simulink model "battery_pack_72v"  (R2020a)
settings: Solver=ode23t  StartTime=0.0  StopTime=5  RelTol=1e-3
libraries: fl_lib x1674, nesl_utility x2
(part 1 of 13)
settings Model: Creator=SIDD N  LastModifiedBy=SIDD N

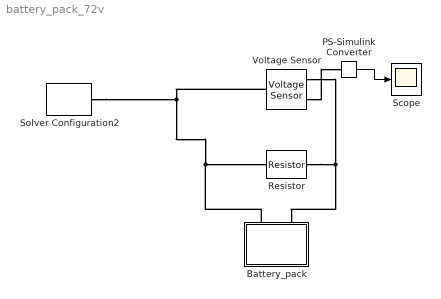
== system battery_pack_72v ==
  Battery_pack : Subsystem
      mask Display: image('$imagefile'); % Use "Edit Image" on toolstrip to change.
  PS-Simulink Converter : nesl_utility/PS-Simulink Converter  PhysicalDomain=network_engine_domain  SubClassName=ps_output  LeftPortType=input  RightPortType=output  PseudoPeriodic=off  Frequencies=[]  Unit=inherit  AffineConversion=off
  Resistor : fl_lib/Electrical/Electrical Elements/Resistor  R=10000 Ohm  i_specify=off  i_priority=None  i=0 A  i_nominal_specify=off  i_nominal_unit=A  i_nominal_value=1  v_specify=off  v_priority=None  v=0 V  v_nominal_specify=off  v_nominal_unit=V  v_nominal_value=1
  Scope : Scope
  Solver Configuration2 : nesl_utility/Solver Configuration  PhysicalDomain=network_engine_domain  SubClassName=solver  LeftPortType=input  RightPortType=generic  Tones=[]  Harmonics=[]  SimulateNoise=off  Profile=off  UseLocalSampling=off  EnableSwitchedLinearOptims=on  FrequencyDomain=off  UseCCode=off  RelTol=0.001  AbsTol=1e-06  MinStep=1e-09  ToWorkspace=off  RevertToSquareIcSolve=off  NumHomotopyIterations=100  PhasorMode=off  PhasorModeNumHarmonics=1  DoDC=off  ResidualTolerance=1e-09  UseLocalSolver=off  LocalSolverChoice=NE_BACKWARD_EULER_ADVANCER  LocalSolverSampleTime=1e-7  DoFixedCost=off  MaxNonlinIter=3  MaxModeIter=2  LinearAlgebra=Sparse  EquationFormulation=NE_TIME_EF  DelaysMemoryBudget=1024  AutomaticFiltering=on  FilteringTimeConstant=0.001  PartitionStorageMethod=AS_NEEDED  PartitionMemoryBudget=1024  PartitionMethod=FAST
  Voltage Sensor : fl_lib/Electrical/Electrical Sensors/Voltage Sensor
  wires:
  PS-Simulink Converter/1 -> Scope/1
  connections:
  Voltage Sensor/RConn1 -- PS-Simulink Converter/LConn1
  Voltage Sensor/LConn1 -- Solver Configuration2/RConn1 -- Battery_pack/LConn1 -- Resistor/LConn1
  Voltage Sensor/RConn2 -- Resistor/RConn1 -- Battery_pack/LConn2

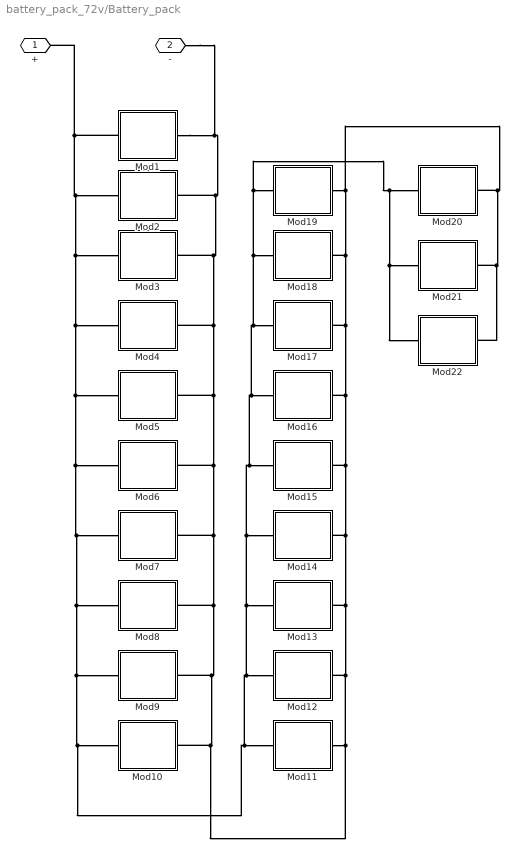
== system battery_pack_72v/Battery_pack ==
  Mod1 : Subsystem
      mask Display: image('C:\Users\SIDD N\Desktop\Screenshot 2020-11-21 19581dwqdq9.png'); % Use "Edit Image" on toolstrip to change.
  Mod10 : Subsystem
      mask Display: image('C:\Users\SIDD N\Desktop\Screenshot 2020-11-21 19581dwqdq9.png'); % Use "Edit Image" on toolstrip to change.
  Mod11 : Subsystem
      mask Display: image('C:\Users\SIDD N\Desktop\Screenshot 2020-11-21 19581dwqdq9.png'); % Use "Edit Image" on toolstrip to change.
  Mod12 : Subsystem
      mask Display: image('C:\Users\SIDD N\Desktop\Screenshot 2020-11-21 19581dwqdq9.png'); % Use "Edit Image" on toolstrip to change.
  Mod13 : Subsystem
      mask Display: image('C:\Users\SIDD N\Desktop\Screenshot 2020-11-21 19581dwqdq9.png'); % Use "Edit Image" on toolstrip to change.
  Mod14 : Subsystem
      mask Display: image('C:\Users\SIDD N\Desktop\Screenshot 2020-11-21 19581dwqdq9.png'); % Use "Edit Image" on toolstrip to change.
  Mod15 : Subsystem
      mask Display: image('C:\Users\SIDD N\Desktop\Screenshot 2020-11-21 19581dwqdq9.png'); % Use "Edit Image" on toolstrip to change.
  Mod16 : Subsystem
      mask Display: image('C:\Users\SIDD N\Desktop\Screenshot 2020-11-21 19581dwqdq9.png'); % Use "Edit Image" on toolstrip to change.
  Mod17 : Subsystem
      mask Display: image('C:\Users\SIDD N\Desktop\Screenshot 2020-11-21 19581dwqdq9.png'); % Use "Edit Image" on toolstrip to change.
  Mod18 : Subsystem
      mask Display: image('C:\Users\SIDD N\Desktop\Screenshot 2020-11-21 19581dwqdq9.png'); % Use "Edit Image" on toolstrip to change.
  Mod19 : Subsystem
      mask Display: image('C:\Users\SIDD N\Desktop\Screenshot 2020-11-21 19581dwqdq9.png'); % Use "Edit Image" on toolstrip to change.
  Mod2 : Subsystem
      mask Display: image('C:\Users\SIDD N\Desktop\Screenshot 2020-11-21 19581dwqdq9.png'); % Use "Edit Image" on toolstrip to change.
  Mod20 : Subsystem
      mask Display: image('C:\Users\SIDD N\Desktop\Screenshot 2020-11-21 19581dwqdq9.png'); % Use "Edit Image" on toolstrip to change.
  Mod21 : Subsystem
      mask Display: image('C:\Users\SIDD N\Desktop\Screenshot 2020-11-21 19581dwqdq9.png'); % Use "Edit Image" on toolstrip to change.
  Mod22 : Subsystem
      mask Display: image('C:\Users\SIDD N\Desktop\Screenshot 2020-11-21 19581dwqdq9.png'); % Use "Edit Image" on toolstrip to change.
  Mod3 : Subsystem
      mask Display: image('C:\Users\SIDD N\Desktop\Screenshot 2020-11-21 19581dwqdq9.png'); % Use "Edit Image" on toolstrip to change.
  Mod4 : Subsystem
      mask Display: image('C:\Users\SIDD N\Desktop\Screenshot 2020-11-21 19581dwqdq9.png'); % Use "Edit Image" on toolstrip to change.
  Mod5 : Subsystem
      mask Display: image('C:\Users\SIDD N\Desktop\Screenshot 2020-11-21 19581dwqdq9.png'); % Use "Edit Image" on toolstrip to change.
  Mod6 : Subsystem
      mask Display: image('C:\Users\SIDD N\Desktop\Screenshot 2020-11-21 19581dwqdq9.png'); % Use "Edit Image" on toolstrip to change.
  Mod7 : Subsystem
      mask Display: image('C:\Users\SIDD N\Desktop\Screenshot 2020-11-21 19581dwqdq9.png'); % Use "Edit Image" on toolstrip to change.
  Mod8 : Subsystem
      mask Display: image('C:\Users\SIDD N\Desktop\Screenshot 2020-11-21 19581dwqdq9.png'); % Use "Edit Image" on toolstrip to change.
  Mod9 : Subsystem
      mask Display: image('C:\Users\SIDD N\Desktop\Screenshot 2020-11-21 19581dwqdq9.png'); % Use "Edit Image" on toolstrip to change.
  + : PMIOPort  Side=Left
  - : PMIOPort  Port=2  Side=Left
  connections:
  Mod19/RConn1 -- Mod12/RConn1 -- Mod11/RConn1 -- Mod10/RConn1 -- Mod9/RConn1 -- Mod6/RConn1 -- Mod4/RConn1 -- Mod3/RConn1 -- -/RConn1 -- Mod1/RConn1 -- Mod2/RConn1 -- Mod5/RConn1 -- Mod7/RConn1 -- Mod8/RConn1 -- Mod13/RConn1 -- Mod14/RConn1 -- Mod15/RConn1 -- Mod16/RConn1 -- Mod17/RConn1 -- Mod18/RConn1 -- Mod22/RConn1 -- Mod21/RConn1 -- Mod20/RConn1
  Mod22/LConn1 -- Mod21/LConn1 -- Mod20/LConn1 -- Mod19/LConn1 -- Mod18/LConn1 -- Mod17/LConn1 -- Mod16/LConn1 -- Mod15/LConn1 -- Mod14/LConn1 -- Mod13/LConn1 -- Mod12/LConn1 -- Mod11/LConn1 -- Mod10/LConn1 -- Mod9/LConn1 -- Mod8/LConn1 -- Mod7/LConn1 -- Mod6/LConn1 -- Mod5/LConn1 -- Mod4/LConn1 -- Mod3/LConn1 -- Mod2/LConn1 -- +/RConn1 -- Mod1/LConn1

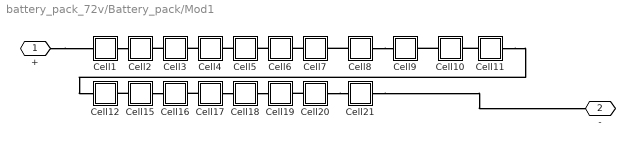
== system battery_pack_72v/Battery_pack/Mod1 ==
  Cell1 : Subsystem
  Cell10 : Subsystem
  Cell11 : Subsystem
  Cell12 : Subsystem
  Cell15 : Subsystem
  Cell16 : Subsystem
  Cell17 : Subsystem
  Cell18 : Subsystem
  Cell19 : Subsystem
  Cell2 : Subsystem
  Cell20 : Subsystem
  Cell21 : Subsystem
  Cell3 : Subsystem
  Cell4 : Subsystem
  Cell5 : Subsystem
  Cell6 : Subsystem
  Cell7 : Subsystem
  Cell8 : Subsystem
  Cell9 : Subsystem
  + : PMIOPort  Side=Left
  - : PMIOPort  Port=2  Side=Right
  connections:
  Cell15/RConn1 -- Cell16/LConn1
  Cell11/LConn1 -- Cell10/RConn1
  Cell8/LConn1 -- Cell7/RConn1
  Cell20/LConn1 -- Cell19/RConn1
  Cell7/LConn1 -- Cell6/RConn1
  Cell17/LConn1 -- Cell16/RConn1
  Cell20/RConn1 -- Cell21/LConn1
  Cell17/RConn1 -- Cell18/LConn1
  Cell3/LConn1 -- Cell2/RConn1
  Cell5/LConn1 -- Cell4/RConn1
  Cell18/RConn1 -- Cell19/LConn1
  Cell8/RConn1 -- Cell9/LConn1
  Cell15/LConn1 -- Cell12/RConn1
  Cell4/LConn1 -- Cell3/RConn1
  Cell11/RConn1 -- Cell12/LConn1
  Cell10/LConn1 -- Cell9/RConn1
  Cell6/LConn1 -- Cell5/RConn1
  Cell1/RConn1 -- Cell2/LConn1
  Cell21/RConn1 -- -/RConn1
  +/RConn1 -- Cell1/LConn1

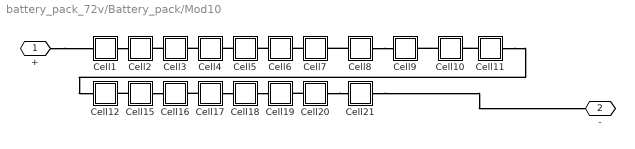
== system battery_pack_72v/Battery_pack/Mod10 ==
  Cell1 : Subsystem
  Cell10 : Subsystem
  Cell11 : Subsystem
  Cell12 : Subsystem
  Cell15 : Subsystem
  Cell16 : Subsystem
  Cell17 : Subsystem
  Cell18 : Subsystem
  Cell19 : Subsystem
  Cell2 : Subsystem
  Cell20 : Subsystem
  Cell21 : Subsystem
  Cell3 : Subsystem
  Cell4 : Subsystem
  Cell5 : Subsystem
  Cell6 : Subsystem
  Cell7 : Subsystem
  Cell8 : Subsystem
  Cell9 : Subsystem
  + : PMIOPort  Side=Left
  - : PMIOPort  Port=2  Side=Right
  connections:
  +/RConn1 -- Cell1/LConn1
  Cell21/RConn1 -- -/RConn1
  Cell1/RConn1 -- Cell2/LConn1
  Cell6/LConn1 -- Cell5/RConn1
  Cell10/LConn1 -- Cell9/RConn1
  Cell11/RConn1 -- Cell12/LConn1
  Cell4/LConn1 -- Cell3/RConn1
  Cell15/LConn1 -- Cell12/RConn1
  Cell8/RConn1 -- Cell9/LConn1
  Cell18/RConn1 -- Cell19/LConn1
  Cell5/LConn1 -- Cell4/RConn1
  Cell3/LConn1 -- Cell2/RConn1
  Cell17/RConn1 -- Cell18/LConn1
  Cell20/RConn1 -- Cell21/LConn1
  Cell17/LConn1 -- Cell16/RConn1
  Cell7/LConn1 -- Cell6/RConn1
  Cell20/LConn1 -- Cell19/RConn1
  Cell8/LConn1 -- Cell7/RConn1
  Cell11/LConn1 -- Cell10/RConn1
  Cell15/RConn1 -- Cell16/LConn1

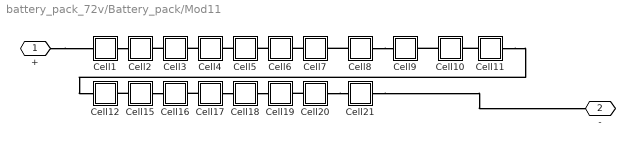
== system battery_pack_72v/Battery_pack/Mod11 ==
  Cell1 : Subsystem
  Cell10 : Subsystem
  Cell11 : Subsystem
  Cell12 : Subsystem
  Cell15 : Subsystem
  Cell16 : Subsystem
  Cell17 : Subsystem
  Cell18 : Subsystem
  Cell19 : Subsystem
  Cell2 : Subsystem
  Cell20 : Subsystem
  Cell21 : Subsystem
  Cell3 : Subsystem
  Cell4 : Subsystem
  Cell5 : Subsystem
  Cell6 : Subsystem
  Cell7 : Subsystem
  Cell8 : Subsystem
  Cell9 : Subsystem
  + : PMIOPort  Side=Left
  - : PMIOPort  Port=2  Side=Right
  connections:
  +/RConn1 -- Cell1/LConn1
  Cell21/RConn1 -- -/RConn1
  Cell1/RConn1 -- Cell2/LConn1
  Cell6/LConn1 -- Cell5/RConn1
  Cell10/LConn1 -- Cell9/RConn1
  Cell11/RConn1 -- Cell12/LConn1
  Cell4/LConn1 -- Cell3/RConn1
  Cell15/LConn1 -- Cell12/RConn1
  Cell8/RConn1 -- Cell9/LConn1
  Cell18/RConn1 -- Cell19/LConn1
  Cell5/LConn1 -- Cell4/RConn1
  Cell3/LConn1 -- Cell2/RConn1
  Cell17/RConn1 -- Cell18/LConn1
  Cell20/RConn1 -- Cell21/LConn1
  Cell17/LConn1 -- Cell16/RConn1
  Cell7/LConn1 -- Cell6/RConn1
  Cell20/LConn1 -- Cell19/RConn1
  Cell8/LConn1 -- Cell7/RConn1
  Cell11/LConn1 -- Cell10/RConn1
  Cell15/RConn1 -- Cell16/LConn1

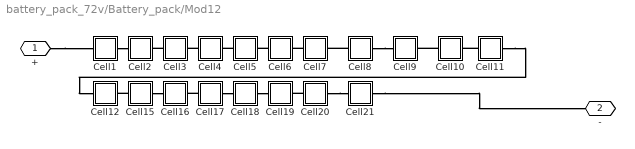
== system battery_pack_72v/Battery_pack/Mod12 ==
  Cell1 : Subsystem
  Cell10 : Subsystem
  Cell11 : Subsystem
  Cell12 : Subsystem
  Cell15 : Subsystem
  Cell16 : Subsystem
  Cell17 : Subsystem
  Cell18 : Subsystem
  Cell19 : Subsystem
  Cell2 : Subsystem
  Cell20 : Subsystem
  Cell21 : Subsystem
  Cell3 : Subsystem
  Cell4 : Subsystem
  Cell5 : Subsystem
  Cell6 : Subsystem
  Cell7 : Subsystem
  Cell8 : Subsystem
  Cell9 : Subsystem
  + : PMIOPort  Side=Left
  - : PMIOPort  Port=2  Side=Right
  connections:
  Cell15/RConn1 -- Cell16/LConn1
  Cell11/LConn1 -- Cell10/RConn1
  Cell8/LConn1 -- Cell7/RConn1
  Cell20/LConn1 -- Cell19/RConn1
  Cell7/LConn1 -- Cell6/RConn1
  Cell17/LConn1 -- Cell16/RConn1
  Cell20/RConn1 -- Cell21/LConn1
  Cell17/RConn1 -- Cell18/LConn1
  Cell3/LConn1 -- Cell2/RConn1
  Cell5/LConn1 -- Cell4/RConn1
  Cell18/RConn1 -- Cell19/LConn1
  Cell8/RConn1 -- Cell9/LConn1
  Cell15/LConn1 -- Cell12/RConn1
  Cell4/LConn1 -- Cell3/RConn1
  Cell11/RConn1 -- Cell12/LConn1
  Cell10/LConn1 -- Cell9/RConn1
  Cell6/LConn1 -- Cell5/RConn1
  Cell1/RConn1 -- Cell2/LConn1
  Cell21/RConn1 -- -/RConn1
  +/RConn1 -- Cell1/LConn1

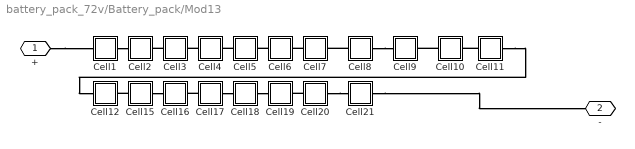
== system battery_pack_72v/Battery_pack/Mod13 ==
  Cell1 : Subsystem
  Cell10 : Subsystem
  Cell11 : Subsystem
  Cell12 : Subsystem
  Cell15 : Subsystem
  Cell16 : Subsystem
  Cell17 : Subsystem
  Cell18 : Subsystem
  Cell19 : Subsystem
  Cell2 : Subsystem
  Cell20 : Subsystem
  Cell21 : Subsystem
  Cell3 : Subsystem
  Cell4 : Subsystem
  Cell5 : Subsystem
  Cell6 : Subsystem
  Cell7 : Subsystem
  Cell8 : Subsystem
  Cell9 : Subsystem
  + : PMIOPort  Side=Left
  - : PMIOPort  Port=2  Side=Right
  connections:
  Cell15/RConn1 -- Cell16/LConn1
  Cell11/LConn1 -- Cell10/RConn1
  Cell8/LConn1 -- Cell7/RConn1
  Cell20/LConn1 -- Cell19/RConn1
  Cell7/LConn1 -- Cell6/RConn1
  Cell17/LConn1 -- Cell16/RConn1
  Cell20/RConn1 -- Cell21/LConn1
  Cell17/RConn1 -- Cell18/LConn1
  Cell3/LConn1 -- Cell2/RConn1
  Cell5/LConn1 -- Cell4/RConn1
  Cell18/RConn1 -- Cell19/LConn1
  Cell8/RConn1 -- Cell9/LConn1
  Cell15/LConn1 -- Cell12/RConn1
  Cell4/LConn1 -- Cell3/RConn1
  Cell11/RConn1 -- Cell12/LConn1
  Cell10/LConn1 -- Cell9/RConn1
  Cell6/LConn1 -- Cell5/RConn1
  Cell1/RConn1 -- Cell2/LConn1
  Cell21/RConn1 -- -/RConn1
  +/RConn1 -- Cell1/LConn1

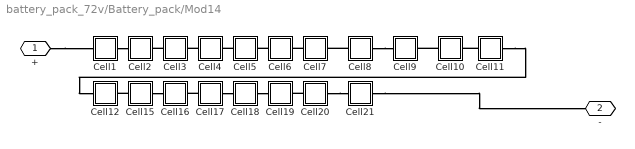
== system battery_pack_72v/Battery_pack/Mod14 ==
  Cell1 : Subsystem
  Cell10 : Subsystem
  Cell11 : Subsystem
  Cell12 : Subsystem
  Cell15 : Subsystem
  Cell16 : Subsystem
  Cell17 : Subsystem
  Cell18 : Subsystem
  Cell19 : Subsystem
  Cell2 : Subsystem
  Cell20 : Subsystem
  Cell21 : Subsystem
  Cell3 : Subsystem
  Cell4 : Subsystem
  Cell5 : Subsystem
  Cell6 : Subsystem
  Cell7 : Subsystem
  Cell8 : Subsystem
  Cell9 : Subsystem
  + : PMIOPort  Side=Left
  - : PMIOPort  Port=2  Side=Right
  connections:
  +/RConn1 -- Cell1/LConn1
  Cell21/RConn1 -- -/RConn1
  Cell1/RConn1 -- Cell2/LConn1
  Cell6/LConn1 -- Cell5/RConn1
  Cell10/LConn1 -- Cell9/RConn1
  Cell11/RConn1 -- Cell12/LConn1
  Cell4/LConn1 -- Cell3/RConn1
  Cell15/LConn1 -- Cell12/RConn1
  Cell8/RConn1 -- Cell9/LConn1
  Cell18/RConn1 -- Cell19/LConn1
  Cell5/LConn1 -- Cell4/RConn1
  Cell3/LConn1 -- Cell2/RConn1
  Cell17/RConn1 -- Cell18/LConn1
  Cell20/RConn1 -- Cell21/LConn1
  Cell17/LConn1 -- Cell16/RConn1
  Cell7/LConn1 -- Cell6/RConn1
  Cell20/LConn1 -- Cell19/RConn1
  Cell8/LConn1 -- Cell7/RConn1
  Cell11/LConn1 -- Cell10/RConn1
  Cell15/RConn1 -- Cell16/LConn1

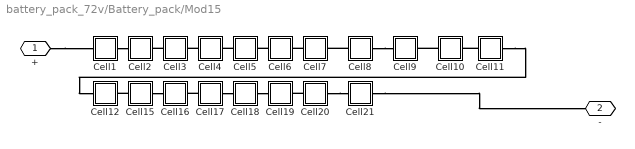
== system battery_pack_72v/Battery_pack/Mod15 ==
  Cell1 : Subsystem
  Cell10 : Subsystem
  Cell11 : Subsystem
  Cell12 : Subsystem
  Cell15 : Subsystem
  Cell16 : Subsystem
  Cell17 : Subsystem
  Cell18 : Subsystem
  Cell19 : Subsystem
  Cell2 : Subsystem
  Cell20 : Subsystem
  Cell21 : Subsystem
  Cell3 : Subsystem
  Cell4 : Subsystem
  Cell5 : Subsystem
  Cell6 : Subsystem
  Cell7 : Subsystem
  Cell8 : Subsystem
  Cell9 : Subsystem
  + : PMIOPort  Side=Left
  - : PMIOPort  Port=2  Side=Right
  connections:
  Cell15/RConn1 -- Cell16/LConn1
  Cell11/LConn1 -- Cell10/RConn1
  Cell8/LConn1 -- Cell7/RConn1
  Cell20/LConn1 -- Cell19/RConn1
  Cell7/LConn1 -- Cell6/RConn1
  Cell17/LConn1 -- Cell16/RConn1
  Cell20/RConn1 -- Cell21/LConn1
  Cell17/RConn1 -- Cell18/LConn1
  Cell3/LConn1 -- Cell2/RConn1
  Cell5/LConn1 -- Cell4/RConn1
  Cell18/RConn1 -- Cell19/LConn1
  Cell8/RConn1 -- Cell9/LConn1
  Cell15/LConn1 -- Cell12/RConn1
  Cell4/LConn1 -- Cell3/RConn1
  Cell11/RConn1 -- Cell12/LConn1
  Cell10/LConn1 -- Cell9/RConn1
  Cell6/LConn1 -- Cell5/RConn1
  Cell1/RConn1 -- Cell2/LConn1
  Cell21/RConn1 -- -/RConn1
  +/RConn1 -- Cell1/LConn1

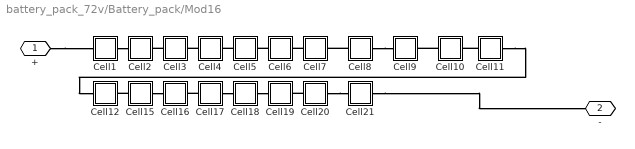
== system battery_pack_72v/Battery_pack/Mod16 ==
  Cell1 : Subsystem
  Cell10 : Subsystem
  Cell11 : Subsystem
  Cell12 : Subsystem
  Cell15 : Subsystem
  Cell16 : Subsystem
  Cell17 : Subsystem
  Cell18 : Subsystem
  Cell19 : Subsystem
  Cell2 : Subsystem
  Cell20 : Subsystem
  Cell21 : Subsystem
  Cell3 : Subsystem
  Cell4 : Subsystem
  Cell5 : Subsystem
  Cell6 : Subsystem
  Cell7 : Subsystem
  Cell8 : Subsystem
  Cell9 : Subsystem
  + : PMIOPort  Side=Left
  - : PMIOPort  Port=2  Side=Right
  connections:
  +/RConn1 -- Cell1/LConn1
  Cell21/RConn1 -- -/RConn1
  Cell1/RConn1 -- Cell2/LConn1
  Cell6/LConn1 -- Cell5/RConn1
  Cell10/LConn1 -- Cell9/RConn1
  Cell11/RConn1 -- Cell12/LConn1
  Cell4/LConn1 -- Cell3/RConn1
  Cell15/LConn1 -- Cell12/RConn1
  Cell8/RConn1 -- Cell9/LConn1
  Cell18/RConn1 -- Cell19/LConn1
  Cell5/LConn1 -- Cell4/RConn1
  Cell3/LConn1 -- Cell2/RConn1
  Cell17/RConn1 -- Cell18/LConn1
  Cell20/RConn1 -- Cell21/LConn1
  Cell17/LConn1 -- Cell16/RConn1
  Cell7/LConn1 -- Cell6/RConn1
  Cell20/LConn1 -- Cell19/RConn1
  Cell8/LConn1 -- Cell7/RConn1
  Cell11/LConn1 -- Cell10/RConn1
  Cell15/RConn1 -- Cell16/LConn1

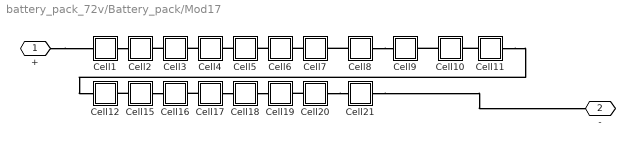
== system battery_pack_72v/Battery_pack/Mod17 ==
  Cell1 : Subsystem
  Cell10 : Subsystem
  Cell11 : Subsystem
  Cell12 : Subsystem
  Cell15 : Subsystem
  Cell16 : Subsystem
  Cell17 : Subsystem
  Cell18 : Subsystem
  Cell19 : Subsystem
  Cell2 : Subsystem
  Cell20 : Subsystem
  Cell21 : Subsystem
  Cell3 : Subsystem
  Cell4 : Subsystem
  Cell5 : Subsystem
  Cell6 : Subsystem
  Cell7 : Subsystem
  Cell8 : Subsystem
  Cell9 : Subsystem
  + : PMIOPort  Side=Left
  - : PMIOPort  Port=2  Side=Right
  connections:
  Cell15/RConn1 -- Cell16/LConn1
  Cell11/LConn1 -- Cell10/RConn1
  Cell8/LConn1 -- Cell7/RConn1
  Cell20/LConn1 -- Cell19/RConn1
  Cell7/LConn1 -- Cell6/RConn1
  Cell17/LConn1 -- Cell16/RConn1
  Cell20/RConn1 -- Cell21/LConn1
  Cell17/RConn1 -- Cell18/LConn1
  Cell3/LConn1 -- Cell2/RConn1
  Cell5/LConn1 -- Cell4/RConn1
  Cell18/RConn1 -- Cell19/LConn1
  Cell8/RConn1 -- Cell9/LConn1
  Cell15/LConn1 -- Cell12/RConn1
  Cell4/LConn1 -- Cell3/RConn1
  Cell11/RConn1 -- Cell12/LConn1
  Cell10/LConn1 -- Cell9/RConn1
  Cell6/LConn1 -- Cell5/RConn1
  Cell1/RConn1 -- Cell2/LConn1
  Cell21/RConn1 -- -/RConn1
  +/RConn1 -- Cell1/LConn1

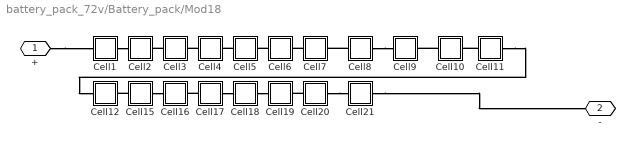
== system battery_pack_72v/Battery_pack/Mod18 ==
  Cell1 : Subsystem
  Cell10 : Subsystem
  Cell11 : Subsystem
  Cell12 : Subsystem
  Cell15 : Subsystem
  Cell16 : Subsystem
  Cell17 : Subsystem
  Cell18 : Subsystem
  Cell19 : Subsystem
  Cell2 : Subsystem
  Cell20 : Subsystem
  Cell21 : Subsystem
  Cell3 : Subsystem
  Cell4 : Subsystem
  Cell5 : Subsystem
  Cell6 : Subsystem
  Cell7 : Subsystem
  Cell8 : Subsystem
  Cell9 : Subsystem
  + : PMIOPort  Side=Left
  - : PMIOPort  Port=2  Side=Right
  connections:
  +/RConn1 -- Cell1/LConn1
  Cell21/RConn1 -- -/RConn1
  Cell1/RConn1 -- Cell2/LConn1
  Cell6/LConn1 -- Cell5/RConn1
  Cell10/LConn1 -- Cell9/RConn1
  Cell11/RConn1 -- Cell12/LConn1
  Cell4/LConn1 -- Cell3/RConn1
  Cell15/LConn1 -- Cell12/RConn1
  Cell8/RConn1 -- Cell9/LConn1
  Cell18/RConn1 -- Cell19/LConn1
  Cell5/LConn1 -- Cell4/RConn1
  Cell3/LConn1 -- Cell2/RConn1
  Cell17/RConn1 -- Cell18/LConn1
  Cell20/RConn1 -- Cell21/LConn1
  Cell17/LConn1 -- Cell16/RConn1
  Cell7/LConn1 -- Cell6/RConn1
  Cell20/LConn1 -- Cell19/RConn1
  Cell8/LConn1 -- Cell7/RConn1
  Cell11/LConn1 -- Cell10/RConn1
  Cell15/RConn1 -- Cell16/LConn1

== system battery_pack_72v/Battery_pack/Mod19 ==
  Cell1 : Subsystem
  Cell10 : Subsystem
  Cell11 : Subsystem
  Cell12 : Subsystem
  Cell15 : Subsystem
  Cell16 : Subsystem
  Cell17 : Subsystem
  Cell18 : Subsystem
  Cell19 : Subsystem
  Cell2 : Subsystem
  Cell20 : Subsystem
  Cell21 : Subsystem
  Cell3 : Subsystem
  Cell4 : Subsystem
  Cell5 : Subsystem
  Cell6 : Subsystem
  Cell7 : Subsystem
  Cell8 : Subsystem
  Cell9 : Subsystem
  + : PMIOPort  Side=Left
  - : PMIOPort  Port=2  Side=Right
  connections:
  Cell15/RConn1 -- Cell16/LConn1
  Cell11/LConn1 -- Cell10/RConn1
  Cell8/LConn1 -- Cell7/RConn1
  Cell20/LConn1 -- Cell19/RConn1
  Cell7/LConn1 -- Cell6/RConn1
  Cell17/LConn1 -- Cell16/RConn1
  Cell20/RConn1 -- Cell21/LConn1
  Cell17/RConn1 -- Cell18/LConn1
  Cell3/LConn1 -- Cell2/RConn1
  Cell5/LConn1 -- Cell4/RConn1
  Cell18/RConn1 -- Cell19/LConn1
  Cell8/RConn1 -- Cell9/LConn1
  Cell15/LConn1 -- Cell12/RConn1
  Cell4/LConn1 -- Cell3/RConn1
  Cell11/RConn1 -- Cell12/LConn1
  Cell10/LConn1 -- Cell9/RConn1
  Cell6/LConn1 -- Cell5/RConn1
  Cell1/RConn1 -- Cell2/LConn1
  Cell21/RConn1 -- -/RConn1
  +/RConn1 -- Cell1/LConn1

== system battery_pack_72v/Battery_pack/Mod2 ==
  Cell1 : Subsystem
  Cell10 : Subsystem
  Cell11 : Subsystem
  Cell12 : Subsystem
  Cell15 : Subsystem
  Cell16 : Subsystem
  Cell17 : Subsystem
  Cell18 : Subsystem
  Cell19 : Subsystem
  Cell2 : Subsystem
  Cell20 : Subsystem
  Cell21 : Subsystem
  Cell3 : Subsystem
  Cell4 : Subsystem
  Cell5 : Subsystem
  Cell6 : Subsystem
  Cell7 : Subsystem
  Cell8 : Subsystem
  Cell9 : Subsystem
  + : PMIOPort  Side=Left
  - : PMIOPort  Port=2  Side=Right
  connections:
  +/RConn1 -- Cell1/LConn1
  Cell21/RConn1 -- -/RConn1
  Cell1/RConn1 -- Cell2/LConn1
  Cell6/LConn1 -- Cell5/RConn1
  Cell10/LConn1 -- Cell9/RConn1
  Cell11/RConn1 -- Cell12/LConn1
  Cell4/LConn1 -- Cell3/RConn1
  Cell15/LConn1 -- Cell12/RConn1
  Cell8/RConn1 -- Cell9/LConn1
  Cell18/RConn1 -- Cell19/LConn1
  Cell5/LConn1 -- Cell4/RConn1
  Cell3/LConn1 -- Cell2/RConn1
  Cell17/RConn1 -- Cell18/LConn1
  Cell20/RConn1 -- Cell21/LConn1
  Cell17/LConn1 -- Cell16/RConn1
  Cell7/LConn1 -- Cell6/RConn1
  Cell20/LConn1 -- Cell19/RConn1
  Cell8/LConn1 -- Cell7/RConn1
  Cell11/LConn1 -- Cell10/RConn1
  Cell15/RConn1 -- Cell16/LConn1

== system battery_pack_72v/Battery_pack/Mod20 ==
  Cell1 : Subsystem
  Cell10 : Subsystem
  Cell11 : Subsystem
  Cell12 : Subsystem
  Cell15 : Subsystem
  Cell16 : Subsystem
  Cell17 : Subsystem
  Cell18 : Subsystem
  Cell19 : Subsystem
  Cell2 : Subsystem
  Cell20 : Subsystem
  Cell21 : Subsystem
  Cell3 : Subsystem
  Cell4 : Subsystem
  Cell5 : Subsystem
  Cell6 : Subsystem
  Cell7 : Subsystem
  Cell8 : Subsystem
  Cell9 : Subsystem
  + : PMIOPort  Side=Left
  - : PMIOPort  Port=2  Side=Right
  connections:
  +/RConn1 -- Cell1/LConn1
  Cell21/RConn1 -- -/RConn1
  Cell1/RConn1 -- Cell2/LConn1
  Cell6/LConn1 -- Cell5/RConn1
  Cell10/LConn1 -- Cell9/RConn1
  Cell11/RConn1 -- Cell12/LConn1
  Cell4/LConn1 -- Cell3/RConn1
  Cell15/LConn1 -- Cell12/RConn1
  Cell8/RConn1 -- Cell9/LConn1
  Cell18/RConn1 -- Cell19/LConn1
  Cell5/LConn1 -- Cell4/RConn1
  Cell3/LConn1 -- Cell2/RConn1
  Cell17/RConn1 -- Cell18/LConn1
  Cell20/RConn1 -- Cell21/LConn1
  Cell17/LConn1 -- Cell16/RConn1
  Cell7/LConn1 -- Cell6/RConn1
  Cell20/LConn1 -- Cell19/RConn1
  Cell8/LConn1 -- Cell7/RConn1
  Cell11/LConn1 -- Cell10/RConn1
  Cell15/RConn1 -- Cell16/LConn1

== system battery_pack_72v/Battery_pack/Mod21 ==
  Cell1 : Subsystem
  Cell10 : Subsystem
  Cell11 : Subsystem
  Cell12 : Subsystem
  Cell15 : Subsystem
  Cell16 : Subsystem
  Cell17 : Subsystem
  Cell18 : Subsystem
  Cell19 : Subsystem
  Cell2 : Subsystem
  Cell20 : Subsystem
  Cell21 : Subsystem
  Cell3 : Subsystem
  Cell4 : Subsystem
  Cell5 : Subsystem
  Cell6 : Subsystem
  Cell7 : Subsystem
  Cell8 : Subsystem
  Cell9 : Subsystem
  + : PMIOPort  Side=Left
  - : PMIOPort  Port=2  Side=Right
  connections:
  Cell15/RConn1 -- Cell16/LConn1
  Cell11/LConn1 -- Cell10/RConn1
  Cell8/LConn1 -- Cell7/RConn1
  Cell20/LConn1 -- Cell19/RConn1
  Cell7/LConn1 -- Cell6/RConn1
  Cell17/LConn1 -- Cell16/RConn1
  Cell20/RConn1 -- Cell21/LConn1
  Cell17/RConn1 -- Cell18/LConn1
  Cell3/LConn1 -- Cell2/RConn1
  Cell5/LConn1 -- Cell4/RConn1
  Cell18/RConn1 -- Cell19/LConn1
  Cell8/RConn1 -- Cell9/LConn1
  Cell15/LConn1 -- Cell12/RConn1
  Cell4/LConn1 -- Cell3/RConn1
  Cell11/RConn1 -- Cell12/LConn1
  Cell10/LConn1 -- Cell9/RConn1
  Cell6/LConn1 -- Cell5/RConn1
  Cell1/RConn1 -- Cell2/LConn1
  Cell21/RConn1 -- -/RConn1
  +/RConn1 -- Cell1/LConn1

== system battery_pack_72v/Battery_pack/Mod22 ==
  Cell1 : Subsystem
  Cell10 : Subsystem
  Cell11 : Subsystem
  Cell12 : Subsystem
  Cell15 : Subsystem
  Cell16 : Subsystem
  Cell17 : Subsystem
  Cell18 : Subsystem
  Cell19 : Subsystem
  Cell2 : Subsystem
  Cell20 : Subsystem
  Cell21 : Subsystem
  Cell3 : Subsystem
  Cell4 : Subsystem
  Cell5 : Subsystem
  Cell6 : Subsystem
  Cell7 : Subsystem
  Cell8 : Subsystem
  Cell9 : Subsystem
  + : PMIOPort  Side=Left
  - : PMIOPort  Port=2  Side=Right
  connections:
  +/RConn1 -- Cell1/LConn1
  Cell21/RConn1 -- -/RConn1
  Cell1/RConn1 -- Cell2/LConn1
  Cell6/LConn1 -- Cell5/RConn1
  Cell10/LConn1 -- Cell9/RConn1
  Cell11/RConn1 -- Cell12/LConn1
  Cell4/LConn1 -- Cell3/RConn1
  Cell15/LConn1 -- Cell12/RConn1
  Cell8/RConn1 -- Cell9/LConn1
  Cell18/RConn1 -- Cell19/LConn1
  Cell5/LConn1 -- Cell4/RConn1
  Cell3/LConn1 -- Cell2/RConn1
  Cell17/RConn1 -- Cell18/LConn1
  Cell20/RConn1 -- Cell21/LConn1
  Cell17/LConn1 -- Cell16/RConn1
  Cell7/LConn1 -- Cell6/RConn1
  Cell20/LConn1 -- Cell19/RConn1
  Cell8/LConn1 -- Cell7/RConn1
  Cell11/LConn1 -- Cell10/RConn1
  Cell15/RConn1 -- Cell16/LConn1

== system battery_pack_72v/Battery_pack/Mod3 ==
  Cell1 : Subsystem
  Cell10 : Subsystem
  Cell11 : Subsystem
  Cell12 : Subsystem
  Cell15 : Subsystem
  Cell16 : Subsystem
  Cell17 : Subsystem
  Cell18 : Subsystem
  Cell19 : Subsystem
  Cell2 : Subsystem
  Cell20 : Subsystem
  Cell21 : Subsystem
  Cell3 : Subsystem
  Cell4 : Subsystem
  Cell5 : Subsystem
  Cell6 : Subsystem
  Cell7 : Subsystem
  Cell8 : Subsystem
  Cell9 : Subsystem
  + : PMIOPort  Side=Left
  - : PMIOPort  Port=2  Side=Right
  connections:
  Cell15/RConn1 -- Cell16/LConn1
  Cell11/LConn1 -- Cell10/RConn1
  Cell8/LConn1 -- Cell7/RConn1
  Cell20/LConn1 -- Cell19/RConn1
  Cell7/LConn1 -- Cell6/RConn1
  Cell17/LConn1 -- Cell16/RConn1
  Cell20/RConn1 -- Cell21/LConn1
  Cell17/RConn1 -- Cell18/LConn1
  Cell3/LConn1 -- Cell2/RConn1
  Cell5/LConn1 -- Cell4/RConn1
  Cell18/RConn1 -- Cell19/LConn1
  Cell8/RConn1 -- Cell9/LConn1
  Cell15/LConn1 -- Cell12/RConn1
  Cell4/LConn1 -- Cell3/RConn1
  Cell11/RConn1 -- Cell12/LConn1
  Cell10/LConn1 -- Cell9/RConn1
  Cell6/LConn1 -- Cell5/RConn1
  Cell1/RConn1 -- Cell2/LConn1
  Cell21/RConn1 -- -/RConn1
  +/RConn1 -- Cell1/LConn1

== system battery_pack_72v/Battery_pack/Mod4 ==
  Cell1 : Subsystem
  Cell10 : Subsystem
  Cell11 : Subsystem
  Cell12 : Subsystem
  Cell15 : Subsystem
  Cell16 : Subsystem
  Cell17 : Subsystem
  Cell18 : Subsystem
  Cell19 : Subsystem
  Cell2 : Subsystem
  Cell20 : Subsystem
  Cell21 : Subsystem
  Cell3 : Subsystem
  Cell4 : Subsystem
  Cell5 : Subsystem
  Cell6 : Subsystem
  Cell7 : Subsystem
  Cell8 : Subsystem
  Cell9 : Subsystem
  + : PMIOPort  Side=Left
  - : PMIOPort  Port=2  Side=Right
  connections:
  +/RConn1 -- Cell1/LConn1
  Cell21/RConn1 -- -/RConn1
  Cell1/RConn1 -- Cell2/LConn1
  Cell6/LConn1 -- Cell5/RConn1
  Cell10/LConn1 -- Cell9/RConn1
  Cell11/RConn1 -- Cell12/LConn1
  Cell4/LConn1 -- Cell3/RConn1
  Cell15/LConn1 -- Cell12/RConn1
  Cell8/RConn1 -- Cell9/LConn1
  Cell18/RConn1 -- Cell19/LConn1
  Cell5/LConn1 -- Cell4/RConn1
  Cell3/LConn1 -- Cell2/RConn1
  Cell17/RConn1 -- Cell18/LConn1
  Cell20/RConn1 -- Cell21/LConn1
  Cell17/LConn1 -- Cell16/RConn1
  Cell7/LConn1 -- Cell6/RConn1
  Cell20/LConn1 -- Cell19/RConn1
  Cell8/LConn1 -- Cell7/RConn1
  Cell11/LConn1 -- Cell10/RConn1
  Cell15/RConn1 -- Cell16/LConn1

== system battery_pack_72v/Battery_pack/Mod5 ==
  Cell1 : Subsystem
  Cell10 : Subsystem
  Cell11 : Subsystem
  Cell12 : Subsystem
  Cell15 : Subsystem
  Cell16 : Subsystem
  Cell17 : Subsystem
  Cell18 : Subsystem
  Cell19 : Subsystem
  Cell2 : Subsystem
  Cell20 : Subsystem
  Cell21 : Subsystem
  Cell3 : Subsystem
  Cell4 : Subsystem
  Cell5 : Subsystem
  Cell6 : Subsystem
  Cell7 : Subsystem
  Cell8 : Subsystem
  Cell9 : Subsystem
  + : PMIOPort  Side=Left
  - : PMIOPort  Port=2  Side=Right
  connections:
  Cell15/RConn1 -- Cell16/LConn1
  Cell11/LConn1 -- Cell10/RConn1
  Cell8/LConn1 -- Cell7/RConn1
  Cell20/LConn1 -- Cell19/RConn1
  Cell7/LConn1 -- Cell6/RConn1
  Cell17/LConn1 -- Cell16/RConn1
  Cell20/RConn1 -- Cell21/LConn1
  Cell17/RConn1 -- Cell18/LConn1
  Cell3/LConn1 -- Cell2/RConn1
  Cell5/LConn1 -- Cell4/RConn1
  Cell18/RConn1 -- Cell19/LConn1
  Cell8/RConn1 -- Cell9/LConn1
  Cell15/LConn1 -- Cell12/RConn1
  Cell4/LConn1 -- Cell3/RConn1
  Cell11/RConn1 -- Cell12/LConn1
  Cell10/LConn1 -- Cell9/RConn1
  Cell6/LConn1 -- Cell5/RConn1
  Cell1/RConn1 -- Cell2/LConn1
  Cell21/RConn1 -- -/RConn1
  +/RConn1 -- Cell1/LConn1

== system battery_pack_72v/Battery_pack/Mod6 ==
  Cell1 : Subsystem
  Cell10 : Subsystem
  Cell11 : Subsystem
  Cell12 : Subsystem
  Cell15 : Subsystem
  Cell16 : Subsystem
  Cell17 : Subsystem
  Cell18 : Subsystem
  Cell19 : Subsystem
  Cell2 : Subsystem
  Cell20 : Subsystem
  Cell21 : Subsystem
  Cell3 : Subsystem
  Cell4 : Subsystem
  Cell5 : Subsystem
  Cell6 : Subsystem
  Cell7 : Subsystem
  Cell8 : Subsystem
  Cell9 : Subsystem
  + : PMIOPort  Side=Left
  - : PMIOPort  Port=2  Side=Right
  connections:
  +/RConn1 -- Cell1/LConn1
  Cell21/RConn1 -- -/RConn1
  Cell1/RConn1 -- Cell2/LConn1
  Cell6/LConn1 -- Cell5/RConn1
  Cell10/LConn1 -- Cell9/RConn1
  Cell11/RConn1 -- Cell12/LConn1
  Cell4/LConn1 -- Cell3/RConn1
  Cell15/LConn1 -- Cell12/RConn1
  Cell8/RConn1 -- Cell9/LConn1
  Cell18/RConn1 -- Cell19/LConn1
  Cell5/LConn1 -- Cell4/RConn1
  Cell3/LConn1 -- Cell2/RConn1
  Cell17/RConn1 -- Cell18/LConn1
  Cell20/RConn1 -- Cell21/LConn1
  Cell17/LConn1 -- Cell16/RConn1
  Cell7/LConn1 -- Cell6/RConn1
  Cell20/LConn1 -- Cell19/RConn1
  Cell8/LConn1 -- Cell7/RConn1
  Cell11/LConn1 -- Cell10/RConn1
  Cell15/RConn1 -- Cell16/LConn1

== system battery_pack_72v/Battery_pack/Mod7 ==
  Cell1 : Subsystem
  Cell10 : Subsystem
  Cell11 : Subsystem
  Cell12 : Subsystem
  Cell15 : Subsystem
  Cell16 : Subsystem
  Cell17 : Subsystem
  Cell18 : Subsystem
  Cell19 : Subsystem
  Cell2 : Subsystem
  Cell20 : Subsystem
  Cell21 : Subsystem
  Cell3 : Subsystem
  Cell4 : Subsystem
  Cell5 : Subsystem
  Cell6 : Subsystem
  Cell7 : Subsystem
  Cell8 : Subsystem
  Cell9 : Subsystem
  + : PMIOPort  Side=Left
  - : PMIOPort  Port=2  Side=Right
  connections:
  Cell15/RConn1 -- Cell16/LConn1
  Cell11/LConn1 -- Cell10/RConn1
  Cell8/LConn1 -- Cell7/RConn1
  Cell20/LConn1 -- Cell19/RConn1
  Cell7/LConn1 -- Cell6/RConn1
  Cell17/LConn1 -- Cell16/RConn1
  Cell20/RConn1 -- Cell21/LConn1
  Cell17/RConn1 -- Cell18/LConn1
  Cell3/LConn1 -- Cell2/RConn1
  Cell5/LConn1 -- Cell4/RConn1
  Cell18/RConn1 -- Cell19/LConn1
  Cell8/RConn1 -- Cell9/LConn1
  Cell15/LConn1 -- Cell12/RConn1
  Cell4/LConn1 -- Cell3/RConn1
  Cell11/RConn1 -- Cell12/LConn1
  Cell10/LConn1 -- Cell9/RConn1
  Cell6/LConn1 -- Cell5/RConn1
  Cell1/RConn1 -- Cell2/LConn1
  Cell21/RConn1 -- -/RConn1
  +/RConn1 -- Cell1/LConn1

== system battery_pack_72v/Battery_pack/Mod8 ==
  Cell1 : Subsystem
  Cell10 : Subsystem
  Cell11 : Subsystem
  Cell12 : Subsystem
  Cell15 : Subsystem
  Cell16 : Subsystem
  Cell17 : Subsystem
  Cell18 : Subsystem
  Cell19 : Subsystem
  Cell2 : Subsystem
  Cell20 : Subsystem
  Cell21 : Subsystem
  Cell3 : Subsystem
  Cell4 : Subsystem
  Cell5 : Subsystem
  Cell6 : Subsystem
  Cell7 : Subsystem
  Cell8 : Subsystem
  Cell9 : Subsystem
  + : PMIOPort  Side=Left
  - : PMIOPort  Port=2  Side=Right
  connections:
  +/RConn1 -- Cell1/LConn1
  Cell21/RConn1 -- -/RConn1
  Cell1/RConn1 -- Cell2/LConn1
  Cell6/LConn1 -- Cell5/RConn1
  Cell10/LConn1 -- Cell9/RConn1
  Cell11/RConn1 -- Cell12/LConn1
  Cell4/LConn1 -- Cell3/RConn1
  Cell15/LConn1 -- Cell12/RConn1
  Cell8/RConn1 -- Cell9/LConn1
  Cell18/RConn1 -- Cell19/LConn1
  Cell5/LConn1 -- Cell4/RConn1
  Cell3/LConn1 -- Cell2/RConn1
  Cell17/RConn1 -- Cell18/LConn1
  Cell20/RConn1 -- Cell21/LConn1
  Cell17/LConn1 -- Cell16/RConn1
  Cell7/LConn1 -- Cell6/RConn1
  Cell20/LConn1 -- Cell19/RConn1
  Cell8/LConn1 -- Cell7/RConn1
  Cell11/LConn1 -- Cell10/RConn1
  Cell15/RConn1 -- Cell16/LConn1

== system battery_pack_72v/Battery_pack/Mod9 ==
  Cell1 : Subsystem
  Cell10 : Subsystem
  Cell11 : Subsystem
  Cell12 : Subsystem
  Cell15 : Subsystem
  Cell16 : Subsystem
  Cell17 : Subsystem
  Cell18 : Subsystem
  Cell19 : Subsystem
  Cell2 : Subsystem
  Cell20 : Subsystem
  Cell21 : Subsystem
  Cell3 : Subsystem
  Cell4 : Subsystem
  Cell5 : Subsystem
  Cell6 : Subsystem
  Cell7 : Subsystem
  Cell8 : Subsystem
  Cell9 : Subsystem
  + : PMIOPort  Side=Left
  - : PMIOPort  Port=2  Side=Right
  connections:
  Cell15/RConn1 -- Cell16/LConn1
  Cell11/LConn1 -- Cell10/RConn1
  Cell8/LConn1 -- Cell7/RConn1
  Cell20/LConn1 -- Cell19/RConn1
  Cell7/LConn1 -- Cell6/RConn1
  Cell17/LConn1 -- Cell16/RConn1
  Cell20/RConn1 -- Cell21/LConn1
  Cell17/RConn1 -- Cell18/LConn1
  Cell3/LConn1 -- Cell2/RConn1
  Cell5/LConn1 -- Cell4/RConn1
  Cell18/RConn1 -- Cell19/LConn1
  Cell8/RConn1 -- Cell9/LConn1
  Cell15/LConn1 -- Cell12/RConn1
  Cell4/LConn1 -- Cell3/RConn1
  Cell11/RConn1 -- Cell12/LConn1
  Cell10/LConn1 -- Cell9/RConn1
  Cell6/LConn1 -- Cell5/RConn1
  Cell1/RConn1 -- Cell2/LConn1
  Cell21/RConn1 -- -/RConn1
  +/RConn1 -- Cell1/LConn1

== system battery_pack_72v/Battery_pack/Mod1/Cell1 ==
  Capacitor : fl_lib/Electrical/Electrical Elements/Capacitor  c=5000 F  r=1e-6 Ohm  g=0 1/Ohm  i_specify=off  i_priority=High  i=0 A  i_nominal_specify=off  i_nominal_unit=A  i_nominal_value=1  v_specify=off  v_priority=High  v=0 V  v_nominal_specify=off  v_nominal_unit=V  v_nominal_value=1  vc_specify=on  vc_priority=High  vc=0 V  vc_nominal_specify=off  vc_nominal_unit=V  vc_nominal_value=1
  DC Voltage Supply : fl_lib/Electrical/Electrical Sources/DC Voltage Source  v0=3.6 V
  Resistor1 : fl_lib/Electrical/Electrical Elements/Resistor  R=0.01 Ohm  i_specify=off  i_priority=High  i=0 A  i_nominal_specify=off  i_nominal_unit=A  i_nominal_value=1  v_specify=off  v_priority=High  v=0 V  v_nominal_specify=off  v_nominal_unit=V  v_nominal_value=1
  Resistor2 : fl_lib/Electrical/Electrical Elements/Resistor  R=0.005 Ohm  i_specify=off  i_priority=High  i=0 A  i_nominal_specify=off  i_nominal_unit=A  i_nominal_value=1  v_specify=off  v_priority=High  v=0 V  v_nominal_specify=off  v_nominal_unit=V  v_nominal_value=1
  + : PMIOPort  Side=Left
  - : PMIOPort  Port=2  Side=Right
  connections:
  Resistor2/LConn1 -- Capacitor/LConn1 -- Resistor1/RConn1
  DC Voltage Supply/RConn1 -- -/RConn1
  Resistor2/RConn1 -- +/RConn1 -- Capacitor/RConn1
  DC Voltage Supply/LConn1 -- Resistor1/LConn1

== system battery_pack_72v/Battery_pack/Mod1/Cell10 ==
  Capacitor : fl_lib/Electrical/Electrical Elements/Capacitor  c=5000 F  r=1e-6 Ohm  g=0 1/Ohm  i_specify=off  i_priority=High  i=0 A  i_nominal_specify=off  i_nominal_unit=A  i_nominal_value=1  v_specify=off  v_priority=High  v=0 V  v_nominal_specify=off  v_nominal_unit=V  v_nominal_value=1  vc_specify=on  vc_priority=High  vc=0 V  vc_nominal_specify=off  vc_nominal_unit=V  vc_nominal_value=1
  DC Voltage Supply : fl_lib/Electrical/Electrical Sources/DC Voltage Source  v0=3.6 V
  Resistor1 : fl_lib/Electrical/Electrical Elements/Resistor  R=0.01 Ohm  i_specify=off  i_priority=High  i=0 A  i_nominal_specify=off  i_nominal_unit=A  i_nominal_value=1  v_specify=off  v_priority=High  v=0 V  v_nominal_specify=off  v_nominal_unit=V  v_nominal_value=1
  Resistor2 : fl_lib/Electrical/Electrical Elements/Resistor  R=0.005 Ohm  i_specify=off  i_priority=High  i=0 A  i_nominal_specify=off  i_nominal_unit=A  i_nominal_value=1  v_specify=off  v_priority=High  v=0 V  v_nominal_specify=off  v_nominal_unit=V  v_nominal_value=1
  + : PMIOPort  Side=Left
  - : PMIOPort  Port=2  Side=Right
  connections:
  DC Voltage Supply/LConn1 -- Resistor1/LConn1
  Capacitor/RConn1 -- +/RConn1 -- Resistor2/RConn1
  DC Voltage Supply/RConn1 -- -/RConn1
  Resistor1/RConn1 -- Capacitor/LConn1 -- Resistor2/LConn1

== system battery_pack_72v/Battery_pack/Mod1/Cell11 ==
  Capacitor : fl_lib/Electrical/Electrical Elements/Capacitor  c=5000 F  r=1e-6 Ohm  g=0 1/Ohm  i_specify=off  i_priority=High  i=0 A  i_nominal_specify=off  i_nominal_unit=A  i_nominal_value=1  v_specify=off  v_priority=High  v=0 V  v_nominal_specify=off  v_nominal_unit=V  v_nominal_value=1  vc_specify=on  vc_priority=High  vc=0 V  vc_nominal_specify=off  vc_nominal_unit=V  vc_nominal_value=1
  DC Voltage Supply : fl_lib/Electrical/Electrical Sources/DC Voltage Source  v0=3.6 V
  Resistor1 : fl_lib/Electrical/Electrical Elements/Resistor  R=0.01 Ohm  i_specify=off  i_priority=High  i=0 A  i_nominal_specify=off  i_nominal_unit=A  i_nominal_value=1  v_specify=off  v_priority=High  v=0 V  v_nominal_specify=off  v_nominal_unit=V  v_nominal_value=1
  Resistor2 : fl_lib/Electrical/Electrical Elements/Resistor  R=0.005 Ohm  i_specify=off  i_priority=High  i=0 A  i_nominal_specify=off  i_nominal_unit=A  i_nominal_value=1  v_specify=off  v_priority=High  v=0 V  v_nominal_specify=off  v_nominal_unit=V  v_nominal_value=1
  + : PMIOPort  Side=Left
  - : PMIOPort  Port=2  Side=Right
  connections:
  Resistor2/LConn1 -- Capacitor/LConn1 -- Resistor1/RConn1
  DC Voltage Supply/RConn1 -- -/RConn1
  Resistor2/RConn1 -- +/RConn1 -- Capacitor/RConn1
  DC Voltage Supply/LConn1 -- Resistor1/LConn1

== system battery_pack_72v/Battery_pack/Mod1/Cell12 ==
  Capacitor : fl_lib/Electrical/Electrical Elements/Capacitor  c=5000 F  r=1e-6 Ohm  g=0 1/Ohm  i_specify=off  i_priority=High  i=0 A  i_nominal_specify=off  i_nominal_unit=A  i_nominal_value=1  v_specify=off  v_priority=High  v=0 V  v_nominal_specify=off  v_nominal_unit=V  v_nominal_value=1  vc_specify=on  vc_priority=High  vc=0 V  vc_nominal_specify=off  vc_nominal_unit=V  vc_nominal_value=1
  DC Voltage Supply : fl_lib/Electrical/Electrical Sources/DC Voltage Source  v0=3.6 V
  Resistor1 : fl_lib/Electrical/Electrical Elements/Resistor  R=0.01 Ohm  i_specify=off  i_priority=High  i=0 A  i_nominal_specify=off  i_nominal_unit=A  i_nominal_value=1  v_specify=off  v_priority=High  v=0 V  v_nominal_specify=off  v_nominal_unit=V  v_nominal_value=1
  Resistor2 : fl_lib/Electrical/Electrical Elements/Resistor  R=0.005 Ohm  i_specify=off  i_priority=High  i=0 A  i_nominal_specify=off  i_nominal_unit=A  i_nominal_value=1  v_specify=off  v_priority=High  v=0 V  v_nominal_specify=off  v_nominal_unit=V  v_nominal_value=1
  + : PMIOPort  Side=Left
  - : PMIOPort  Port=2  Side=Right
  connections:
  DC Voltage Supply/LConn1 -- Resistor1/LConn1
  Capacitor/RConn1 -- +/RConn1 -- Resistor2/RConn1
  DC Voltage Supply/RConn1 -- -/RConn1
  Resistor1/RConn1 -- Capacitor/LConn1 -- Resistor2/LConn1

== system battery_pack_72v/Battery_pack/Mod1/Cell15 ==
  Capacitor : fl_lib/Electrical/Electrical Elements/Capacitor  c=5000 F  r=1e-6 Ohm  g=0 1/Ohm  i_specify=off  i_priority=High  i=0 A  i_nominal_specify=off  i_nominal_unit=A  i_nominal_value=1  v_specify=off  v_priority=High  v=0 V  v_nominal_specify=off  v_nominal_unit=V  v_nominal_value=1  vc_specify=on  vc_priority=High  vc=0 V  vc_nominal_specify=off  vc_nominal_unit=V  vc_nominal_value=1
  DC Voltage Supply : fl_lib/Electrical/Electrical Sources/DC Voltage Source  v0=3.6 V
  Resistor1 : fl_lib/Electrical/Electrical Elements/Resistor  R=0.01 Ohm  i_specify=off  i_priority=High  i=0 A  i_nominal_specify=off  i_nominal_unit=A  i_nominal_value=1  v_specify=off  v_priority=High  v=0 V  v_nominal_specify=off  v_nominal_unit=V  v_nominal_value=1
  Resistor2 : fl_lib/Electrical/Electrical Elements/Resistor  R=0.005 Ohm  i_specify=off  i_priority=High  i=0 A  i_nominal_specify=off  i_nominal_unit=A  i_nominal_value=1  v_specify=off  v_priority=High  v=0 V  v_nominal_specify=off  v_nominal_unit=V  v_nominal_value=1
  + : PMIOPort  Side=Left
  - : PMIOPort  Port=2  Side=Right
  connections:
  Resistor2/LConn1 -- Capacitor/LConn1 -- Resistor1/RConn1
  DC Voltage Supply/RConn1 -- -/RConn1
  Resistor2/RConn1 -- +/RConn1 -- Capacitor/RConn1
  DC Voltage Supply/LConn1 -- Resistor1/LConn1

== system battery_pack_72v/Battery_pack/Mod1/Cell16 ==
  Capacitor : fl_lib/Electrical/Electrical Elements/Capacitor  c=5000 F  r=1e-6 Ohm  g=0 1/Ohm  i_specify=off  i_priority=High  i=0 A  i_nominal_specify=off  i_nominal_unit=A  i_nominal_value=1  v_specify=off  v_priority=High  v=0 V  v_nominal_specify=off  v_nominal_unit=V  v_nominal_value=1  vc_specify=on  vc_priority=High  vc=0 V  vc_nominal_specify=off  vc_nominal_unit=V  vc_nominal_value=1
  DC Voltage Supply : fl_lib/Electrical/Electrical Sources/DC Voltage Source  v0=3.6 V
  Resistor1 : fl_lib/Electrical/Electrical Elements/Resistor  R=0.01 Ohm  i_specify=off  i_priority=High  i=0 A  i_nominal_specify=off  i_nominal_unit=A  i_nominal_value=1  v_specify=off  v_priority=High  v=0 V  v_nominal_specify=off  v_nominal_unit=V  v_nominal_value=1
  Resistor2 : fl_lib/Electrical/Electrical Elements/Resistor  R=0.005 Ohm  i_specify=off  i_priority=High  i=0 A  i_nominal_specify=off  i_nominal_unit=A  i_nominal_value=1  v_specify=off  v_priority=High  v=0 V  v_nominal_specify=off  v_nominal_unit=V  v_nominal_value=1
  + : PMIOPort  Side=Left
  - : PMIOPort  Port=2  Side=Right
  connections:
  DC Voltage Supply/LConn1 -- Resistor1/LConn1
  Capacitor/RConn1 -- +/RConn1 -- Resistor2/RConn1
  DC Voltage Supply/RConn1 -- -/RConn1
  Resistor1/RConn1 -- Capacitor/LConn1 -- Resistor2/LConn1

== system battery_pack_72v/Battery_pack/Mod1/Cell17 ==
  Capacitor : fl_lib/Electrical/Electrical Elements/Capacitor  c=5000 F  r=1e-6 Ohm  g=0 1/Ohm  i_specify=off  i_priority=High  i=0 A  i_nominal_specify=off  i_nominal_unit=A  i_nominal_value=1  v_specify=off  v_priority=High  v=0 V  v_nominal_specify=off  v_nominal_unit=V  v_nominal_value=1  vc_specify=on  vc_priority=High  vc=0 V  vc_nominal_specify=off  vc_nominal_unit=V  vc_nominal_value=1
  DC Voltage Supply : fl_lib/Electrical/Electrical Sources/DC Voltage Source  v0=3.6 V
  Resistor1 : fl_lib/Electrical/Electrical Elements/Resistor  R=0.01 Ohm  i_specify=off  i_priority=High  i=0 A  i_nominal_specify=off  i_nominal_unit=A  i_nominal_value=1  v_specify=off  v_priority=High  v=0 V  v_nominal_specify=off  v_nominal_unit=V  v_nominal_value=1
  Resistor2 : fl_lib/Electrical/Electrical Elements/Resistor  R=0.005 Ohm  i_specify=off  i_priority=High  i=0 A  i_nominal_specify=off  i_nominal_unit=A  i_nominal_value=1  v_specify=off  v_priority=High  v=0 V  v_nominal_specify=off  v_nominal_unit=V  v_nominal_value=1
  + : PMIOPort  Side=Left
  - : PMIOPort  Port=2  Side=Right
  connections:
  Resistor2/LConn1 -- Capacitor/LConn1 -- Resistor1/RConn1
  DC Voltage Supply/RConn1 -- -/RConn1
  Resistor2/RConn1 -- +/RConn1 -- Capacitor/RConn1
  DC Voltage Supply/LConn1 -- Resistor1/LConn1

== system battery_pack_72v/Battery_pack/Mod1/Cell18 ==
  Capacitor : fl_lib/Electrical/Electrical Elements/Capacitor  c=5000 F  r=1e-6 Ohm  g=0 1/Ohm  i_specify=off  i_priority=High  i=0 A  i_nominal_specify=off  i_nominal_unit=A  i_nominal_value=1  v_specify=off  v_priority=High  v=0 V  v_nominal_specify=off  v_nominal_unit=V  v_nominal_value=1  vc_specify=on  vc_priority=High  vc=0 V  vc_nominal_specify=off  vc_nominal_unit=V  vc_nominal_value=1
  DC Voltage Supply : fl_lib/Electrical/Electrical Sources/DC Voltage Source  v0=3.6 V
  Resistor1 : fl_lib/Electrical/Electrical Elements/Resistor  R=0.01 Ohm  i_specify=off  i_priority=High  i=0 A  i_nominal_specify=off  i_nominal_unit=A  i_nominal_value=1  v_specify=off  v_priority=High  v=0 V  v_nominal_specify=off  v_nominal_unit=V  v_nominal_value=1
  Resistor2 : fl_lib/Electrical/Electrical Elements/Resistor  R=0.005 Ohm  i_specify=off  i_priority=High  i=0 A  i_nominal_specify=off  i_nominal_unit=A  i_nominal_value=1  v_specify=off  v_priority=High  v=0 V  v_nominal_specify=off  v_nominal_unit=V  v_nominal_value=1
  + : PMIOPort  Side=Left
  - : PMIOPort  Port=2  Side=Right
  connections:
  DC Voltage Supply/LConn1 -- Resistor1/LConn1
  Capacitor/RConn1 -- +/RConn1 -- Resistor2/RConn1
  DC Voltage Supply/RConn1 -- -/RConn1
  Resistor1/RConn1 -- Capacitor/LConn1 -- Resistor2/LConn1

== system battery_pack_72v/Battery_pack/Mod1/Cell19 ==
  Capacitor : fl_lib/Electrical/Electrical Elements/Capacitor  c=5000 F  r=1e-6 Ohm  g=0 1/Ohm  i_specify=off  i_priority=High  i=0 A  i_nominal_specify=off  i_nominal_unit=A  i_nominal_value=1  v_specify=off  v_priority=High  v=0 V  v_nominal_specify=off  v_nominal_unit=V  v_nominal_value=1  vc_specify=on  vc_priority=High  vc=0 V  vc_nominal_specify=off  vc_nominal_unit=V  vc_nominal_value=1
  DC Voltage Supply : fl_lib/Electrical/Electrical Sources/DC Voltage Source  v0=3.6 V
  Resistor1 : fl_lib/Electrical/Electrical Elements/Resistor  R=0.01 Ohm  i_specify=off  i_priority=High  i=0 A  i_nominal_specify=off  i_nominal_unit=A  i_nominal_value=1  v_specify=off  v_priority=High  v=0 V  v_nominal_specify=off  v_nominal_unit=V  v_nominal_value=1
  Resistor2 : fl_lib/Electrical/Electrical Elements/Resistor  R=0.005 Ohm  i_specify=off  i_priority=High  i=0 A  i_nominal_specify=off  i_nominal_unit=A  i_nominal_value=1  v_specify=off  v_priority=High  v=0 V  v_nominal_specify=off  v_nominal_unit=V  v_nominal_value=1
  + : PMIOPort  Side=Left
  - : PMIOPort  Port=2  Side=Right
  connections:
  Resistor2/LConn1 -- Capacitor/LConn1 -- Resistor1/RConn1
  DC Voltage Supply/RConn1 -- -/RConn1
  Resistor2/RConn1 -- +/RConn1 -- Capacitor/RConn1
  DC Voltage Supply/LConn1 -- Resistor1/LConn1

== system battery_pack_72v/Battery_pack/Mod1/Cell2 ==
  Capacitor : fl_lib/Electrical/Electrical Elements/Capacitor  c=5000 F  r=1e-6 Ohm  g=0 1/Ohm  i_specify=off  i_priority=High  i=0 A  i_nominal_specify=off  i_nominal_unit=A  i_nominal_value=1  v_specify=off  v_priority=High  v=0 V  v_nominal_specify=off  v_nominal_unit=V  v_nominal_value=1  vc_specify=on  vc_priority=High  vc=0 V  vc_nominal_specify=off  vc_nominal_unit=V  vc_nominal_value=1
  DC Voltage Supply : fl_lib/Electrical/Electrical Sources/DC Voltage Source  v0=3.6 V
  Resistor1 : fl_lib/Electrical/Electrical Elements/Resistor  R=0.01 Ohm  i_specify=off  i_priority=High  i=0 A  i_nominal_specify=off  i_nominal_unit=A  i_nominal_value=1  v_specify=off  v_priority=High  v=0 V  v_nominal_specify=off  v_nominal_unit=V  v_nominal_value=1
  Resistor2 : fl_lib/Electrical/Electrical Elements/Resistor  R=0.005 Ohm  i_specify=off  i_priority=High  i=0 A  i_nominal_specify=off  i_nominal_unit=A  i_nominal_value=1  v_specify=off  v_priority=High  v=0 V  v_nominal_specify=off  v_nominal_unit=V  v_nominal_value=1
  + : PMIOPort  Side=Left
  - : PMIOPort  Port=2  Side=Right
  connections:
  DC Voltage Supply/LConn1 -- Resistor1/LConn1
  Capacitor/RConn1 -- +/RConn1 -- Resistor2/RConn1
  DC Voltage Supply/RConn1 -- -/RConn1
  Resistor1/RConn1 -- Capacitor/LConn1 -- Resistor2/LConn1

== system battery_pack_72v/Battery_pack/Mod1/Cell20 ==
  Capacitor : fl_lib/Electrical/Electrical Elements/Capacitor  c=5000 F  r=1e-6 Ohm  g=0 1/Ohm  i_specify=off  i_priority=High  i=0 A  i_nominal_specify=off  i_nominal_unit=A  i_nominal_value=1  v_specify=off  v_priority=High  v=0 V  v_nominal_specify=off  v_nominal_unit=V  v_nominal_value=1  vc_specify=on  vc_priority=High  vc=0 V  vc_nominal_specify=off  vc_nominal_unit=V  vc_nominal_value=1
  DC Voltage Supply : fl_lib/Electrical/Electrical Sources/DC Voltage Source  v0=3.6 V
  Resistor1 : fl_lib/Electrical/Electrical Elements/Resistor  R=0.01 Ohm  i_specify=off  i_priority=High  i=0 A  i_nominal_specify=off  i_nominal_unit=A  i_nominal_value=1  v_specify=off  v_priority=High  v=0 V  v_nominal_specify=off  v_nominal_unit=V  v_nominal_value=1
  Resistor2 : fl_lib/Electrical/Electrical Elements/Resistor  R=0.005 Ohm  i_specify=off  i_priority=High  i=0 A  i_nominal_specify=off  i_nominal_unit=A  i_nominal_value=1  v_specify=off  v_priority=High  v=0 V  v_nominal_specify=off  v_nominal_unit=V  v_nominal_value=1
  + : PMIOPort  Side=Left
  - : PMIOPort  Port=2  Side=Right
  connections:
  DC Voltage Supply/LConn1 -- Resistor1/LConn1
  Capacitor/RConn1 -- +/RConn1 -- Resistor2/RConn1
  DC Voltage Supply/RConn1 -- -/RConn1
  Resistor1/RConn1 -- Capacitor/LConn1 -- Resistor2/LConn1

== system battery_pack_72v/Battery_pack/Mod1/Cell21 ==
  Capacitor : fl_lib/Electrical/Electrical Elements/Capacitor  c=5000 F  r=1e-6 Ohm  g=0 1/Ohm  i_specify=off  i_priority=High  i=0 A  i_nominal_specify=off  i_nominal_unit=A  i_nominal_value=1  v_specify=off  v_priority=High  v=0 V  v_nominal_specify=off  v_nominal_unit=V  v_nominal_value=1  vc_specify=on  vc_priority=High  vc=0 V  vc_nominal_specify=off  vc_nominal_unit=V  vc_nominal_value=1
  DC Voltage Supply : fl_lib/Electrical/Electrical Sources/DC Voltage Source  v0=3.6 V
  Resistor1 : fl_lib/Electrical/Electrical Elements/Resistor  R=0.01 Ohm  i_specify=off  i_priority=High  i=0 A  i_nominal_specify=off  i_nominal_unit=A  i_nominal_value=1  v_specify=off  v_priority=High  v=0 V  v_nominal_specify=off  v_nominal_unit=V  v_nominal_value=1
  Resistor2 : fl_lib/Electrical/Electrical Elements/Resistor  R=0.005 Ohm  i_specify=off  i_priority=High  i=0 A  i_nominal_specify=off  i_nominal_unit=A  i_nominal_value=1  v_specify=off  v_priority=High  v=0 V  v_nominal_specify=off  v_nominal_unit=V  v_nominal_value=1
  + : PMIOPort  Side=Left
  - : PMIOPort  Port=2  Side=Right
  connections:
  Resistor2/LConn1 -- Capacitor/LConn1 -- Resistor1/RConn1
  DC Voltage Supply/RConn1 -- -/RConn1
  Resistor2/RConn1 -- +/RConn1 -- Capacitor/RConn1
  DC Voltage Supply/LConn1 -- Resistor1/LConn1

== system battery_pack_72v/Battery_pack/Mod1/Cell3 ==
  Capacitor : fl_lib/Electrical/Electrical Elements/Capacitor  c=5000 F  r=1e-6 Ohm  g=0 1/Ohm  i_specify=off  i_priority=High  i=0 A  i_nominal_specify=off  i_nominal_unit=A  i_nominal_value=1  v_specify=off  v_priority=High  v=0 V  v_nominal_specify=off  v_nominal_unit=V  v_nominal_value=1  vc_specify=on  vc_priority=High  vc=0 V  vc_nominal_specify=off  vc_nominal_unit=V  vc_nominal_value=1
  DC Voltage Supply : fl_lib/Electrical/Electrical Sources/DC Voltage Source  v0=3.6 V
  Resistor1 : fl_lib/Electrical/Electrical Elements/Resistor  R=0.01 Ohm  i_specify=off  i_priority=High  i=0 A  i_nominal_specify=off  i_nominal_unit=A  i_nominal_value=1  v_specify=off  v_priority=High  v=0 V  v_nominal_specify=off  v_nominal_unit=V  v_nominal_value=1
  Resistor2 : fl_lib/Electrical/Electrical Elements/Resistor  R=0.005 Ohm  i_specify=off  i_priority=High  i=0 A  i_nominal_specify=off  i_nominal_unit=A  i_nominal_value=1  v_specify=off  v_priority=High  v=0 V  v_nominal_specify=off  v_nominal_unit=V  v_nominal_value=1
  + : PMIOPort  Side=Left
  - : PMIOPort  Port=2  Side=Right
  connections:
  Resistor2/LConn1 -- Capacitor/LConn1 -- Resistor1/RConn1
  DC Voltage Supply/RConn1 -- -/RConn1
  Resistor2/RConn1 -- +/RConn1 -- Capacitor/RConn1
  DC Voltage Supply/LConn1 -- Resistor1/LConn1
